simulink model "Point3S_test4"  (R2023a)
settings: Solver=VariableStepAuto  StartTime=0.0  StopTime=10.0  RelTol=1e-3
settings Model: Creator=bjmyn  LastModifiedBy=bjmyn
settings DebuggingCC: AlgebraicLoopMsg=none

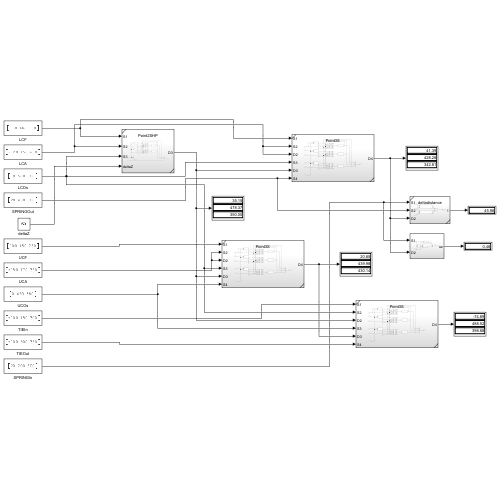
[thumbnail: Simulink's stored preview of the top-level diagram]
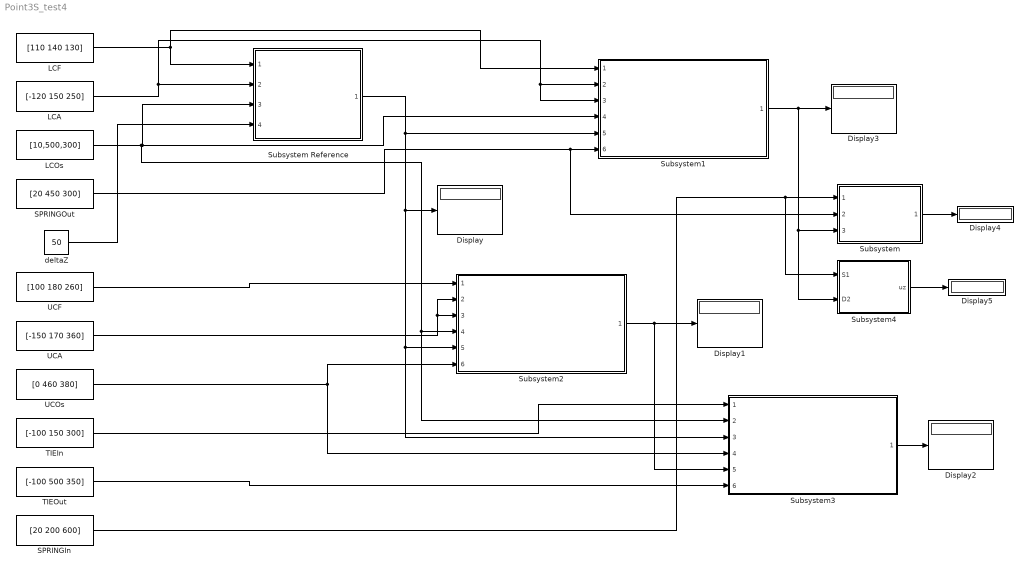
== system Point3S_test4 ==
  Display{,1..5} (6 alike) : Display
      settings: Format=bank
  LCA : Constant  Value=[-120 150 250]
  LCF : Constant  Value=[110 140 130]
  LCOs : Constant  Value=[10,500,300]
  SPRINGIn : Constant  Value=[20 200 600]
  SPRINGOut : Constant  Value=[20 450 300]
  Subsystem : Subsystem  ReferencedSubsystem=deltadistance
  Subsystem Reference : Subsystem  ReferencedSubsystem=Point2SHP
  Subsystem1 : Subsystem  ReferencedSubsystem=Point3S
  Subsystem2 : Subsystem  ReferencedSubsystem=Point3S
  Subsystem3 : Subsystem  ReferencedSubsystem=Point3S
  Subsystem4 : Subsystem
  TIEIn : Constant  Value=[-100 150 300]
  TIEOut : Constant  Value=[-100 500 350]
  UCA : Constant  Value=[-150 170 360]
  UCF : Constant  Value=[100 180 260]
  UCOs : Constant  Value=[0 460 380]
  deltaZ : Constant  Value=50
  wires:
  LCOs/1 -> Subsystem1/4, Subsystem Reference/3, Subsystem2/4, Subsystem3/2
  deltaZ/1 -> Subsystem Reference/4
  LCA/1 -> Subsystem1/3, Subsystem1/2, Subsystem Reference/2
  LCF/1 -> Subsystem1/1, Subsystem Reference/1
  Subsystem Reference/1 -> Subsystem1/5, Display/1, Subsystem2/5, Subsystem3/3
  UCF/1 -> Subsystem2/1
  UCA/1 -> Subsystem2/2, Subsystem2/3
  UCOs/1 -> Subsystem2/6, Subsystem3/4
  Subsystem2/1 -> Subsystem3/5, Display1/1
  TIEIn/1 -> Subsystem3/1
  TIEOut/1 -> Subsystem3/6
  Subsystem3/1 -> Display2/1
  SPRINGOut/1 -> Subsystem/2, Subsystem1/6
  Subsystem1/1 -> Subsystem4/2(D2), Subsystem/3, Display3/1
  SPRINGIn/1 -> Subsystem4/1(S1), Subsystem/1
  Subsystem/1 -> Display4/1
  Subsystem4/1(uz) -> Display5/1

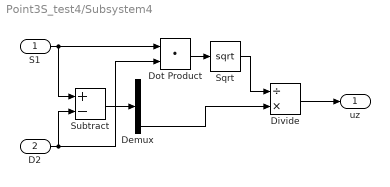
== system Point3S_test4/Subsystem4 ==
  S1 : Inport
  D2 : Inport  Port=2
  Demux : Demux  Outputs=3
  Divide : Product  Inputs=/*
  Dot Product : DotProduct  OutDataTypeStr=Inherit: Inherit via internal rule
  Sqrt : Sqrt
  Subtract : Sum  Inputs=+-
  uz : Outport
  wires:
  S1/1 -> Subtract/1, Dot Product/1
  D2/1 -> Subtract/2, Dot Product/2
  Dot Product/1 -> Sqrt/1
  Divide/1 -> uz/1
  Sqrt/1 -> Divide/1
  Subtract/1 -> Demux/1
  Demux/3 -> Divide/2
